simulink model "NonIsotropicEx"  (R2015a)
settings: Solver=FixedStepDiscrete  StartTime=0.0  StopTime=tsim  FixedStep=dt  RelTol=1e-3
values from neighbouring files (symbols this model uses):
  Cp2d = Cp*ones(length(y0),length(x))    [run_NonIsotropicEx.m]
  hb = 0.035    [run_NonIsotropicEx.m]
  hl = 0.035    [run_NonIsotropicEx.m]
  hr = 0.035    [run_NonIsotropicEx.m]
  ht = 0.035    [run_NonIsotropicEx.m]
  k2dx = k2*ones(length(y0),length(x))    [run_NonIsotropicEx.m]
  k2dy = k1*ones(length(y0),length(x))    [run_NonIsotropicEx.m]
  m = length(y0)    [run_NonIsotropicEx.m]
  n = length(x)    [run_NonIsotropicEx.m]
  rho2d = rho*ones(length(y0),length(x))    [run_NonIsotropicEx.m]
  Tb = 700    [run_NonIsotropicEx.m]
  Tl = 700    [run_NonIsotropicEx.m]
  Tr = 700    [run_NonIsotropicEx.m]
  Tt = 700    [run_NonIsotropicEx.m]
libraries: lib_Conduction_2DCondADI x1
settings Model: Creator=jlkratz  LastModifiedBy=jlkratz

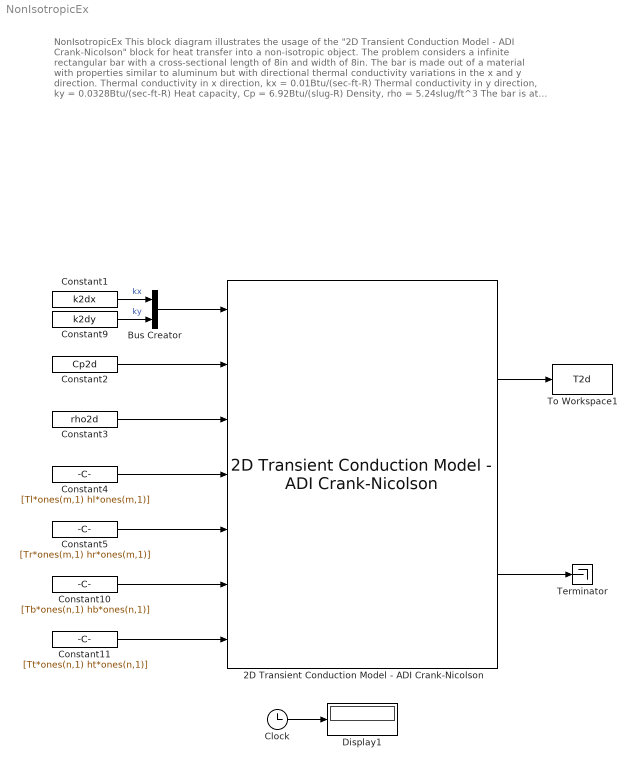
== system NonIsotropicEx ==
  note: NonIsotropicEx
      |
      | This block diagram illustrates the usage of the "2D Transient Conduction Model - ADI Crank-Nicolson" block
      | for heat transfer into a non-isotropic object.
      |
      | The problem considers a infinite rectangular bar with a cross-sectional length of 8in and width of 8in. The bar is made
      | out of a material with properties similar to aluminum but with directional thermal conductivity variations in the x and
      | y direction.
      | Thermal conductivity in x direction, kx = 0.01Btu/(sec-ft-R)
      | Thermal conductivity in y direction, ky = 0.0328Btu/(sec-ft-R)
      | Heat capacity, Cp = 6.92Btu/(slug-R)
      | Density, rho = 5.24slug/ft^3
      | The bar is at an initial temperature of 550R throughout. It is heated on all sides by convection via a fluid with a
      | temperature of 700R and a heat transfer coefficient of 0.035Btu/(sec-ft^2-R)
  2D Transient Conduction Model - ADI Crank-Nicolson : lib_Conduction_2DCondADI/2D Transient Conduction Model - ADI Crank-Nicolson  T0_M=T02d  dt_M=dt  x_M=x  y_M=y0  shape_M=Planar in both directions  convL_M=on  radL_M=off  condL_M=off  convR_M=on  radR_M=off  condR_M=off  convB_M=on  radB_M=off  condB_M=off  convT_M=on  radT_M=off  condT_M=off  BN_M=double(gcb)
  Bus Creator : BusCreator  Inputs=2
  Clock : Clock
  Constant1 : Constant  Value=k2dx
  Constant10 : Constant  Value=[Tb*ones(n,1) hb*ones(n,1)]
  Constant11 : Constant  Value=[Tt*ones(n,1) ht*ones(n,1)]
  Constant2 : Constant  Value=Cp2d
  Constant3 : Constant  Value=rho2d
  Constant4 : Constant  Value=[Tl*ones(m,1) hl*ones(m,1)]
  Constant5 : Constant  Value=[Tr*ones(m,1) hr*ones(m,1)]
  Constant9 : Constant  Value=k2dy
  Display1 : Display
  Terminator : Terminator
  To Workspace1 : ToWorkspace  VariableName=T2d  SaveFormat=Timeseries  SampleTime=-1
  wires:
  Constant1/1 -> Bus Creator/1  "kx"
  Constant9/1 -> Bus Creator/2  "ky"
  Bus Creator/1 -> 2D Transient Conduction Model - ADI Crank-Nicolson/1
  Constant2/1 -> 2D Transient Conduction Model - ADI Crank-Nicolson/2
  Constant3/1 -> 2D Transient Conduction Model - ADI Crank-Nicolson/3
  Constant11/1 -> 2D Transient Conduction Model - ADI Crank-Nicolson/7
  Constant10/1 -> 2D Transient Conduction Model - ADI Crank-Nicolson/6
  2D Transient Conduction Model - ADI Crank-Nicolson/1 -> To Workspace1/1
  2D Transient Conduction Model - ADI Crank-Nicolson/2 -> Terminator/1
  Constant4/1 -> 2D Transient Conduction Model - ADI Crank-Nicolson/4
  Constant5/1 -> 2D Transient Conduction Model - ADI Crank-Nicolson/5
  Clock/1 -> Display1/1
